simulink model "drone_model_advanced"  (R2024b)
settings: Solver=VariableStepAuto  StartTime=0.0  StopTime=10.0  RelTol=1e-3
undefined symbols (not defined in the file or in its folder): b, d, g, J_r, J_xx, J_yy, J_zz, K_dx, K_dy, K_dz, K_LQR, l, m, X0
settings Model: Creator=andit  LastModifiedBy=andit

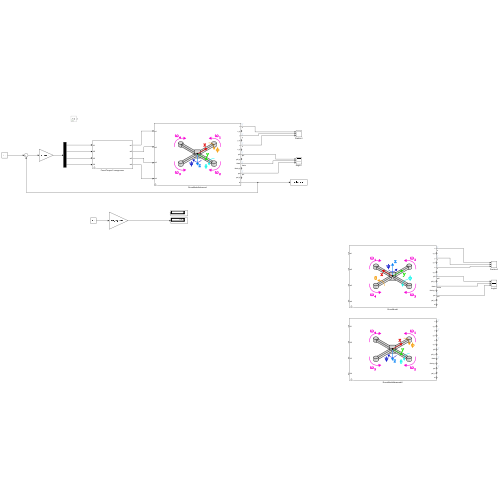
[thumbnail: Simulink's stored preview of the top-level diagram]
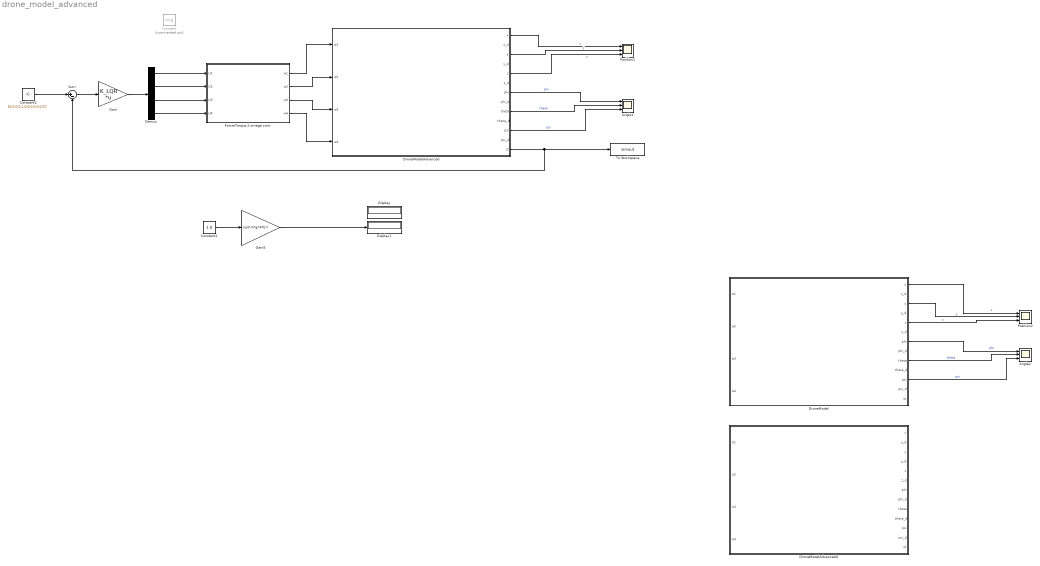
== system drone_model_advanced ==
  Angle1 : Scope  NumInputPorts=3
  Angle2 : Scope  NumInputPorts=3
  Constant : Constant  Commented=on  Value=m*g
  Constant1 : Constant  Value=1.0
  Constant2 : Constant  Value=[0,0,0,0,1,0,0,0,0,0,0,0]'
  Demux : Demux
  Display : Display
  Display1 : Display
  DroneModel : Subsystem  mask{m=m, g=g, l=l, I_xx=J_xx, I_yy=J_yy, I_zz=J_zz, J_r=J_r, b=b, d=d}
      mask prompts: m "mass"; l "length from rotor"; J_r "Motor Inertia J_r"; b "Thrust factor b"; d "Drag factor d"
      mask DialogControl THETA Prompt: Principle Moments of Inertia
      mask DialogControl PROPELLER Prompt: Propeller Coefficients
  DroneModelAdvanced : Subsystem  mask{m=m, g=g, l=l, I_xx=J_xx, I_yy=J_yy, I_zz=J_zz, J_r=J_r, b=b, d=d, K_dx=K_dx, K_dy=K_dy, K_dz=K_dz, X0=X0}
      mask prompts: m "mass"; l "length from rotor"; J_r "Motor Inertia J_r"; b "Thrust factor b"; d "Drag factor d"; K_dx "Drag coeff. drone x"; K_dy "Drag coeff. drone y"; K_dz "Drag coeff. drone z"; X0 "Initial conditions"
      mask DialogControl THETA Prompt: Principle Moments of Inertia
      mask DialogControl PROPELLER Prompt: Propeller Coefficients
      mask DialogControl dronedrag Prompt: Drone Drag Coefficients
  DroneModelAdvancedU : Subsystem  mask{m=m, g=g, l=l, I_xx=J_xx, I_yy=J_yy, I_zz=J_zz, J_r=J_r, b=b, d=d, K_dx=K_dx, K_dy=K_dy, K_dz=K_dz}
      mask prompts: m "mass"; l "length from rotor"; J_r "Motor Inertia J_r"; b "Thrust factor b"; d "Drag factor d"; K_dx "Drag coeff. drone x"; K_dy "Drag coeff. drone y"; K_dz "Drag coeff. drone z"
      mask DialogControl THETA Prompt: Principle Moments of Inertia
      mask DialogControl PROPELLER Prompt: Propeller Coefficients
      mask DialogControl dronedrag Prompt: Drone Drag Coefficients
  Force/Torque 2 omega conv : Subsystem  mask{b=b, d=d}
      mask prompts: b "Thrust factor b"; d "Drag factor d"
      mask DialogControl PROPELLER Prompt: Propeller Coefficients
  Gain : Gain  Gain=K_LQR  Multiplication=Matrix(K*u)
  Gain5 : Gain  Gain=sqrt(m*g/(4*b))
  Position1 : Scope  NumInputPorts=3
  Position2 : Scope  NumInputPorts=3
  Sum : Sum  Inputs=|+-
  To Workspace : ToWorkspace  VariableName=simout  SaveFormat=Timeseries  SampleTime=-1
  wires:
  Constant1/1 -> Gain5/1
  DroneModelAdvanced/1(x) -> Position1/1  "x"
  DroneModelAdvanced/3(y) -> Position1/2  "y"
  DroneModelAdvanced/5(z) -> Position1/3  "z"
  DroneModelAdvanced/7(phi) -> Angle1/1  "phi"
  DroneModelAdvanced/9(theta) -> Angle1/2  "theta"
  DroneModelAdvanced/11(psi) -> Angle1/3  "psi"
  DroneModelAdvanced/13(st) -> Sum/2, To Workspace/1
  DroneModel/1(x) -> Position2/1  "x"
  DroneModel/3(y) -> Position2/2  "y"
  DroneModel/5(z) -> Position2/3  "z"
  DroneModel/7(phi) -> Angle2/1  "phi"
  DroneModel/9(theta) -> Angle2/2  "theta"
  DroneModel/11(psi) -> Angle2/3  "psi"
  Gain5/1 -> Display1/1
  Force/Torque 2 omega conv/1(w1) -> DroneModelAdvanced/1(w1)
  Force/Torque 2 omega conv/2(w2) -> DroneModelAdvanced/2(w2)
  Force/Torque 2 omega conv/3(w3) -> DroneModelAdvanced/3(w3)
  Force/Torque 2 omega conv/4(w4) -> DroneModelAdvanced/4(w4)
  Demux/4 -> Force/Torque 2 omega conv/4(U4)
  Demux/3 -> Force/Torque 2 omega conv/3(U3)
  Demux/2 -> Force/Torque 2 omega conv/2(U2)
  Demux/1 -> Force/Torque 2 omega conv/1(U1)
  Gain/1 -> Demux/1
  Sum/1 -> Gain/1
  Constant2/1 -> Sum/1

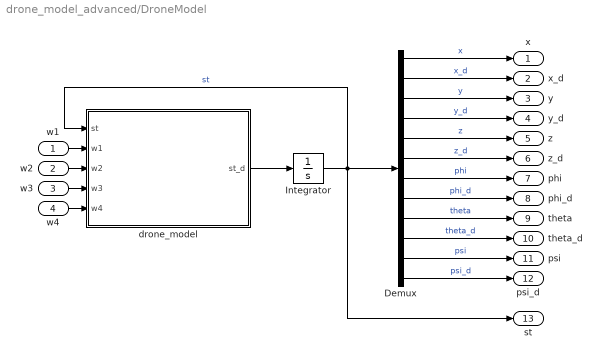
== system drone_model_advanced/DroneModel ==
  w1 : Inport
  w2 : Inport  Port=2
  w3 : Inport  Port=3
  w4 : Inport  Port=4
  Demux : Demux  Outputs=12
  Integrator : Integrator  InitialCondition=zeros(12,1)
  drone_model : MATLAB Function  TreatAsAtomicUnit=on
  x : Outport
  x_d : Outport  Port=2
  y : Outport  Port=3
  y_d : Outport  Port=4
  z : Outport  Port=5
  z_d : Outport  Port=6
  phi : Outport  Port=7
  phi_d : Outport  Port=8
  theta : Outport  Port=9
  theta_d : Outport  Port=10
  psi : Outport  Port=11
  psi_d : Outport  Port=12
  st : Outport  Port=13
  wires:
  drone_model/1(st_d) -> Integrator/1
  Demux/9 -> theta/1  "theta"
  w4/1 -> drone_model/5(w4)
  Integrator/1 -> st/1, Demux/1, drone_model/1(st)  "st"
  w3/1 -> drone_model/4(w3)
  Demux/7 -> phi/1  "phi"
  w2/1 -> drone_model/3(w2)
  w1/1 -> drone_model/2(w1)
  Demux/3 -> y/1  "y"
  Demux/11 -> psi/1  "psi"
  Demux/10 -> theta_d/1  "theta_d"
  Demux/2 -> x_d/1  "x_d"
  Demux/12 -> psi_d/1  "psi_d"
  Demux/6 -> z_d/1  "z_d"
  Demux/1 -> x/1  "x"
  Demux/8 -> phi_d/1  "phi_d"
  Demux/4 -> y_d/1  "y_d"
  Demux/5 -> z/1  "z"

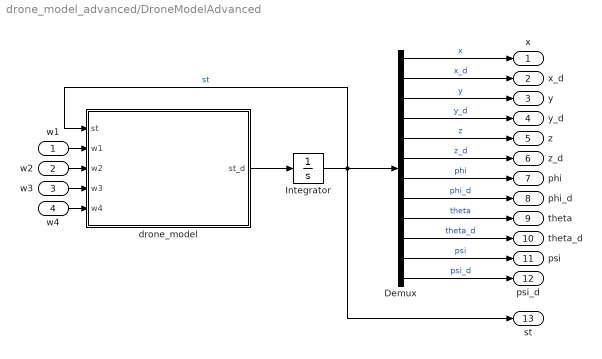
== system drone_model_advanced/DroneModelAdvanced ==
  w1 : Inport
  w2 : Inport  Port=2
  w3 : Inport  Port=3
  w4 : Inport  Port=4
  Demux : Demux  Outputs=12
  Integrator : Integrator  InitialCondition=X0
  drone_model : MATLAB Function  TreatAsAtomicUnit=on
  x : Outport
  x_d : Outport  Port=2
  y : Outport  Port=3
  y_d : Outport  Port=4
  z : Outport  Port=5
  z_d : Outport  Port=6
  phi : Outport  Port=7
  phi_d : Outport  Port=8
  theta : Outport  Port=9
  theta_d : Outport  Port=10
  psi : Outport  Port=11
  psi_d : Outport  Port=12
  st : Outport  Port=13
  wires:
  drone_model/1(st_d) -> Integrator/1
  Demux/9 -> theta/1  "theta"
  w4/1 -> drone_model/5(w4)
  Integrator/1 -> st/1, Demux/1, drone_model/1(st)  "st"
  w3/1 -> drone_model/4(w3)
  Demux/7 -> phi/1  "phi"
  w2/1 -> drone_model/3(w2)
  w1/1 -> drone_model/2(w1)
  Demux/3 -> y/1  "y"
  Demux/11 -> psi/1  "psi"
  Demux/10 -> theta_d/1  "theta_d"
  Demux/2 -> x_d/1  "x_d"
  Demux/12 -> psi_d/1  "psi_d"
  Demux/6 -> z_d/1  "z_d"
  Demux/1 -> x/1  "x"
  Demux/8 -> phi_d/1  "phi_d"
  Demux/4 -> y_d/1  "y_d"
  Demux/5 -> z/1  "z"

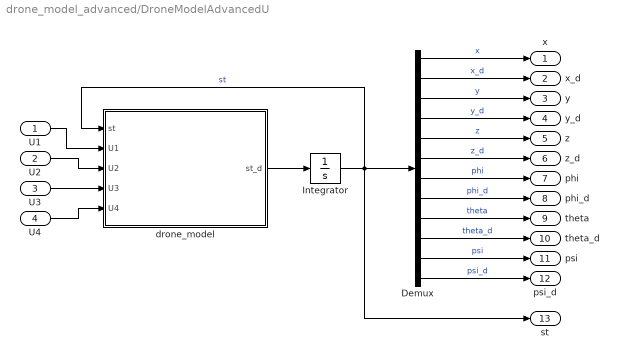
== system drone_model_advanced/DroneModelAdvancedU ==
  U1 : Inport
  U2 : Inport  Port=2
  U3 : Inport  Port=3
  U4 : Inport  Port=4
  Demux : Demux  Outputs=12
  Integrator : Integrator  InitialCondition=zeros(12,1)
  drone_model : MATLAB Function  TreatAsAtomicUnit=on
  x : Outport
  x_d : Outport  Port=2
  y : Outport  Port=3
  y_d : Outport  Port=4
  z : Outport  Port=5
  z_d : Outport  Port=6
  phi : Outport  Port=7
  phi_d : Outport  Port=8
  theta : Outport  Port=9
  theta_d : Outport  Port=10
  psi : Outport  Port=11
  psi_d : Outport  Port=12
  st : Outport  Port=13
  wires:
  drone_model/1(st_d) -> Integrator/1
  Demux/9 -> theta/1  "theta"
  U4/1 -> drone_model/5(U4)
  Integrator/1 -> st/1, Demux/1, drone_model/1(st)  "st"
  U3/1 -> drone_model/4(U3)
  Demux/7 -> phi/1  "phi"
  U2/1 -> drone_model/3(U2)
  U1/1 -> drone_model/2(U1)
  Demux/3 -> y/1  "y"
  Demux/11 -> psi/1  "psi"
  Demux/10 -> theta_d/1  "theta_d"
  Demux/2 -> x_d/1  "x_d"
  Demux/12 -> psi_d/1  "psi_d"
  Demux/6 -> z_d/1  "z_d"
  Demux/1 -> x/1  "x"
  Demux/8 -> phi_d/1  "phi_d"
  Demux/4 -> y_d/1  "y_d"
  Demux/5 -> z/1  "z"

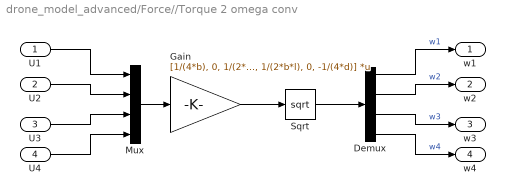
== system drone_model_advanced/Force//Torque 2 omega conv ==
  U1 : Inport
  U2 : Inport  Port=2
  U3 : Inport  Port=3
  U4 : Inport  Port=4
  Demux : Demux
  Gain : Gain  Gain=|  Multiplication=Matrix(K*u) (u vector)
      | [1/(4*b), 0, 1/(2*b*l),  1/(4*d); 1/(4*b), -1/(2*b*l), 0, -1/(4*d);
      | 1/(4*b), 0, -1/(2*b*l), 1/(4*d);
      | 1/(4*b), 1/(2*b*l), 0, -1/(4*d)]
  Mux : Mux
  Sqrt : Sqrt  OutputSignalType=real
  w1 : Outport
  w2 : Outport  Port=2
  w3 : Outport  Port=3
  w4 : Outport  Port=4
  wires:
  Mux/1 -> Gain/1
  Gain/1 -> Sqrt/1
  Sqrt/1 -> Demux/1
  U1/1 -> Mux/1
  U2/1 -> Mux/2
  Demux/4 -> w4/1  "w4"
  Demux/1 -> w1/1  "w1"
  U4/1 -> Mux/4
  Demux/3 -> w3/1  "w3"
  Demux/2 -> w2/1  "w2"
  U3/1 -> Mux/3

== matlab function drone_model_advanced/DroneModel/drone_model ==
  data: st input; st_d output; w1 input; w2 input; w3 input; w4 input; m parameter; g parameter; l parameter; I_xx parameter; I_yy parameter; I_zz parameter; J_r parameter; b parameter; d parameter
function st_d = drone_model(st, w1, w2, w3, w4, m, g, l, I_xx, I_yy, I_zz, J_r, b, d)

% st = [x, x_d, y, y_d, z, z_d, phi, phi_d, theta, theta_d, psi, psi_d]

phi     = st(7);    phi_d   = st(8);
theta   = st(9);    theta_d = st(10);
psi     = st(11);   psi_d   = st(12);

U1 = b*(w1^2 + w2^2 + w3^2 + w4^2);     % total thrust
U2 = b*(w4^2 - w2^2);                   % Force diff for Roll
U3 = b*(w3^2 - w1^2);                   % Force diff for Pitch
U4 = d*(w2^2 + w4^2 - w1^2 - w3^2);     % Drag torque for Yaw
Omega = w1 - w2 + w3 - w4;              % Residual rotor speed

x_dd = 1/m * (cos(phi)*sin(theta)*cos(psi) - sin(phi)*sin(psi))*U1;
y_dd = 1/m * (cos(phi)*sin(theta)*sin(psi) + sin(phi)*cos(psi))*U1;
z_dd = -g + 1/m * (cos(phi)*cos(theta))*U1;

phi_dd = 1/I_xx * (theta_d*psi_d*(I_zz-I_yy) - J_r*theta_d*Omega + l*U2);
theta_dd = 1/I_yy * (phi_d*psi_d*(I_xx-I_zz) + J_r*phi_d*Omega + l*U3);
psi_dd = 1/I_zz * (phi_d*theta_d*(I_yy-I_xx) + U4);

st_d = [st(2); x_dd; ...            % x_d, x_dd
        st(4); y_dd; ...            % y_d, y_dd
        st(6); z_dd; ...            % z_d, z_dd
        st(8); phi_dd; ...          % phi_d, phi_dd
        st(10); theta_dd; ...       % theta_d, theta_dd
        st(12); psi_dd];            % psi_d, psi_dd

== matlab function drone_model_advanced/DroneModelAdvanced/drone_model ==
  data: st input; st_d output; w1 input; w2 input; w3 input; w4 input; m parameter; g parameter; l parameter; I_xx parameter; I_yy parameter; I_zz parameter; J_r parameter; b parameter; d parameter; K_dx parameter; K_dy parameter; K_dz parameter
function st_d = drone_model(st, w1, w2, w3, w4, m, g, l, I_xx, I_yy, I_zz, J_r, b, d, K_dx, K_dy, K_dz)

% st = [x, x_d, y, y_d, z, z_d, phi, phi_d, theta, theta_d, psi, psi_d]
% motors = [w1, w2, w3, w4]

x_d = st(2); y_d = st(4); z_d = st(6);
phi = st(7); phi_d = st(8);
theta = st(9); theta_d = st(10);
psi = st(11); psi_d = st(12);

Omega = w1-w2+w3-w4;
FT_b = b * (w1^2+w2^2+w3^2+w4^2);

p = phi_d - sin(theta) * psi_d;
q = cos(phi) * theta_d + sin(phi) * cos(theta) * psi_d;
r = -sin(phi) * theta_d + cos(phi) * cos(theta) * psi_d;

x_dd = (1/m) * (-(cos(phi)*cos(psi)*sin(theta) + sin(phi)*sin(psi))*FT_b - K_dx*x_d);
y_dd = (1/m) * (-(cos(phi)*sin(psi)*sin(theta) - cos(psi)*sin(phi))*FT_b - K_dy*y_d);
z_dd = (1/m) * (-(cos(phi)*cos(theta))*FT_b - K_dz*z_d) + g;

phi_dd   = (1/I_xx) * ((I_yy - I_zz)*q*r - J_r*q*Omega + l*b*(w4^2 - w2^2));
theta_dd = (1/I_yy) * ((I_zz - I_xx)*p*r + J_r*p*Omega + l*b*(w1^2 - w3^2));
psi_dd   = (1/I_zz) * ((I_xx - I_yy)*p*q + d*(w1^2 - w2^2 + w3^2 - w4^2));

st_d = [st(2); x_dd; ...
        st(4); y_dd; ...
        st(6); z_dd; ...
        st(8); phi_dd; ...
        st(10); theta_dd; ...
        st(12); psi_dd];

== matlab function drone_model_advanced/DroneModelAdvancedU/drone_model ==
  data: st input; st_d output; U1 input; U2 input; U3 input; U4 input; m parameter; g parameter; l parameter; I_xx parameter; I_yy parameter; I_zz parameter; J_r parameter; K_dx parameter; K_dy parameter; K_dz parameter
function st_d = drone_model(st, U1, U2, U3, U4, m, g, l, I_xx, I_yy, I_zz, J_r, K_dx, K_dy, K_dz)

% st = [x, x_d, y, y_d, z, z_d, phi, phi_d, theta, theta_d, psi, psi_d]
% motors = [w1, w2, w3, w4]

x_d = st(2); y_d = st(4); z_d = st(6);
phi = st(7); phi_d = st(8);
theta = st(9); theta_d = st(10);
psi = st(11); psi_d = st(12);

Omega = 0;

p = phi_d - sin(theta) * psi_d;
q = cos(phi) * theta_d + sin(phi) * cos(theta) * psi_d;
r = -sin(phi) * theta_d + cos(phi) * cos(theta) * psi_d;

x_dd = (1/m) * (-(cos(phi)*cos(psi)*sin(theta) + sin(phi)*sin(psi))*U1 - K_dx*x_d);
y_dd = (1/m) * (-(cos(phi)*sin(psi)*sin(theta) - cos(psi)*sin(phi))*U1 - K_dy*y_d);
z_dd = (1/m) * (-(cos(phi)*cos(theta))*U1 - K_dz*z_d) + g;

phi_dd   = (1/I_xx) * ((I_yy - I_zz)*q*r - J_r*q*Omega + l*U2);
theta_dd = (1/I_yy) * ((I_zz - I_xx)*p*r + J_r*p*Omega + l*U3);
psi_dd   = (1/I_zz) * ((I_xx - I_yy)*p*q + U4);

st_d = [st(2); x_dd; ...
        st(4); y_dd; ...
        st(6); z_dd; ...
        st(8); phi_dd; ...
        st(10); theta_dd; ...
        st(12); psi_dd];
